simulink model "DR_Throughput_Model"  (R2026a)
settings: Solver=VariableStepAuto  StopTime=8
settings Model: Creator=SHIVANYA SALES  LastModifiedBy=SHIVANYA SALES

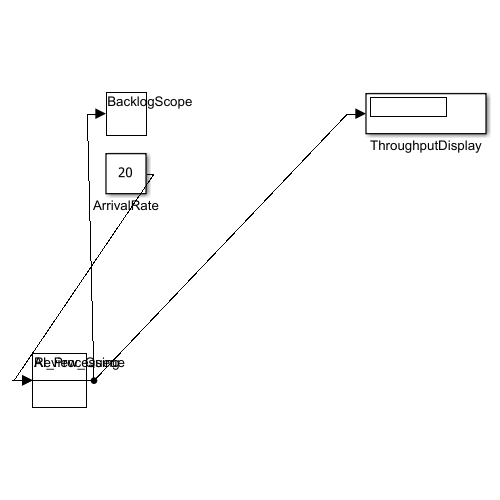
[thumbnail: Simulink's stored preview of the top-level diagram]
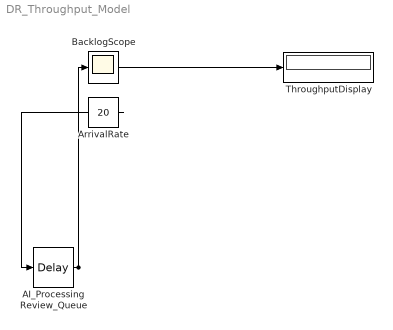
== system DR_Throughput_Model ==
  AI_Processing : TransportDelay  DelayTime=2.5
  ArrivalRate : Constant  Value=20
  BacklogScope : Scope
  Review_Queue : TransportDelay  DelayTime=105
  ThroughputDisplay : Display
  wires:
  ArrivalRate/1 -> AI_Processing/1
  AI_Processing/1 -> Review_Queue/1
  Review_Queue/1 -> BacklogScope/1, ThroughputDisplay/1
